simulink model "verify_Reynolds_mdl"  (R2013b)
settings: Solver=VariableStepDiscrete  StartTime=0.0  StopTime=10.0  MaxStep=0.1  RelTol=1e-3
libraries: carnot x2
settings Model: Creator=drhf  LastModifiedBy=drhf
settings OptimizationCC: ExpressionDepthLimit=2147483647
settings DebuggingCC: StateNameClashWarn=warning
settings GRTTargetCC: CombineOutputUpdateFcns=off  GRTInterface=on

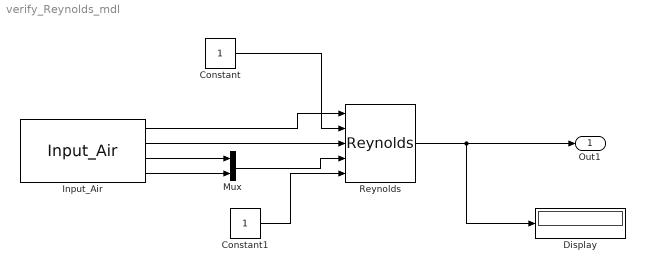
== system verify_Reynolds_mdl ==
  Constant : Constant
  Constant1 : Constant
  Display : Display
  Input_Air : carnot/Basic/Material_Properties/Input_Air  T=0  p=1e5  x=0.0
  Mux : Mux  Inputs=2
  Reynolds : carnot/Basic/Hydraulics/Reynolds
  Out1 : Outport
  wires:
  Input_Air/2 -> Reynolds/3
  Input_Air/1 -> Reynolds/1
  Input_Air/4 -> Mux/2
  Input_Air/3 -> Mux/1
  Reynolds/1 -> Out1/1, Display/1
  Constant/1 -> Reynolds/2
  Mux/1 -> Reynolds/4
  Constant1/1 -> Reynolds/5
